simulink model "read_values_1"  (R2018b)
settings: Solver=VariableStepAuto  StartTime=0.0  StopTime=10.0  RelTol=1e-3
settings Model: Creator=binoythomas  LastModifiedBy=binoythomas

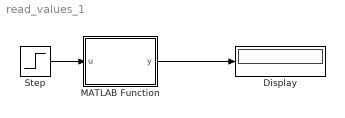
== system read_values_1 ==
  Display : Display
  MATLAB Function : MATLAB Function  TreatAsAtomicUnit=on
  Step : Step  SampleTime=0
  wires:
  MATLAB Function/1(y) -> Display/1
  Step/1 -> MATLAB Function/1(u)

== matlab function read_values_1/MATLAB Function ==
  data: u input; y output
function y = fcn(u)
myev3=legoev3('USB');
ls_read=readInputDeviceREADY_RAW(myev3,2,0,1);
   
y = ls_read;
